simulink model "base_closed_loop_model"  (R2017a)
settings: Solver=ode23  StartTime=0.0  StopTime=5  FixedStep=0.01  MaxStep=0.01  MinStep=0.0001  RelTol=1e-5  AbsTol=1e-6  EnableMultiTasking=on
libraries: simulink x1
settings Model: Creator=cpmcclel  LastModifiedBy=s6bae
settings SolverCC: MaxConsecutiveMinStep=1000  ZeroCrossAlgorithm=Adaptive
settings DataIOCC: LimitDataPoints=on  SaveFormat=Array
settings OptimizationCC: LifeSpan=inf
settings DebuggingCC: SolverPrmCheckMsg=warning  SFUnexpectedBacktrackingDiag=warning  SFNoUnconditionalDefaultTransitionDiag=warning  SFExecutionAtInitializationDiag=none
settings HardwareCC: ProdBitPerPointer=32  ProdBitPerSizeT=32  ProdBitPerPtrDiffT=32  ProdLargestAtomicFloat=None  ProdIntDivRoundTo=Undefined  ProdEndianess=Unspecified  ProdWordSize=32  ProdHWDeviceType=32-bit Generic
settings ModelReferenceCC: PropagateSignalLabelsOutOfModel=off
settings GRTTargetCC: TargetLangStandard=C89/C90 (ANSI)  GeneratePreprocessorConditionals=Disable all
settings ConfigComp: CovMetricSettings=dw  CovHtmlReporting=on  CovSaveCumulativeToWorkspaceVar=on  CovSaveSingleToWorkspaceVar=on  CovExternalEMLEnable=off  CovSFcnEnable=off

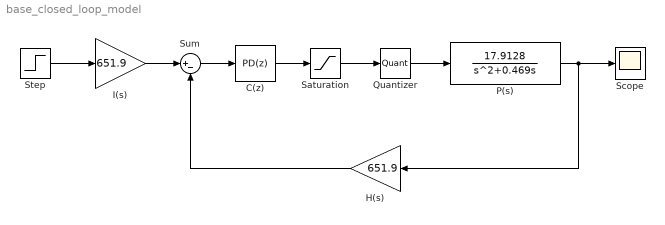
== system base_closed_loop_model ==
  C(z) : simulink/Continuous/PID Controller  Controller=PD  TimeDomain=Discrete-time  SampleTime=0.0159  IntegratorMethod=Forward Euler  FilterMethod=Backward Euler  Form=Parallel  UseFilter=on  ControllerParametersSource=internal  P=0.02773998321  I=64.3  D=0.0025374  N=790.0763  InitialConditionSource=internal  InitialConditionForIntegrator=0  InitialConditionForFilter=0  ExternalReset=none  LimitOutput=off  UpperSaturationLimit=inf  LowerSaturationLimit=-inf  LinearizeAsGain=on  AntiWindupMode=clamping  Kb=1  TrackingMode=off  Kt=1  PParamMin=[]  PParamMax=[]  IParamMin=[]  IParamMax=[]  DParamMin=[]  DParamMax=[]  NParamMin=[]  NParamMax=[]  KbParamMin=[]  KbParamMax=[]  KtParamMin=[]  KtParamMax=[]  POutMin=[]  POutMax=[]  IOutMin=[]  IOutMax=[]  DOutMin=[]  DOutMax=[]  NOutMin=[]  NOutMax=[]  KbOutMin=[]  KbOutMax=[]  KtOutMin=[]  KtOutMax=[]  IntegratorOutMin=[]  IntegratorOutMax=[]  FilterOutMin=[]  FilterOutMax=[]  SumOutMin=[]  SumOutMax=[]  SumI1OutMin=[]  SumI1OutMax=[]  SumI2OutMin=[]  SumI2OutMax=[]  SumI3OutMin=[]  SumI3OutMax=[]  SumDOutMin=[]  SumDOutMax=[]  SaturationOutMin=[]  SaturationOutMax=[]  IntegratorContinuousStateAttributes=''  IntegratorStateMustResolveToSignalObject=off  IntegratorRTWStateStorageClass=Auto  FilterContinuousStateAttributes=''  FilterStateMustResolveToSignalObject=off  FilterRTWStateStorageClass=Auto  DifferentiatorICPrevScaledInput=0  DifferentiatorOutMin=[]  DifferentiatorOutMax=[]  InitialConditionSetting=State (most efficient)
  H(s) : Gain  Gain=651.9
  I(s) : Gain  Gain=651.9
  P(s) : TransferFcn  Numerator=[17.9128]  Denominator=[1 0.469 0]
  Quantizer : Quantizer  QuantizationInterval=12/1024
  Saturation : Saturate  UpperLimit=12  LowerLimit=-12
  Scope : Scope
  Step : Step  Time=0
  Sum : Sum  Inputs=|+-
  wires:
  Step/1 -> I(s)/1
  Sum/1 -> C(z)/1
  Saturation/1 -> Quantizer/1
  C(z)/1 -> Saturation/1
  Quantizer/1 -> P(s)/1
  H(s)/1 -> Sum/2
  I(s)/1 -> Sum/1
  P(s)/1 -> Scope/1, H(s)/1
